simulink library "halout"  (R2021b)
settings: Solver=VariableStepAuto  StartTime=0.0  StopTime=10.0  RelTol=1e-3
undefined symbols (not defined in the file): C_TASK_5MS_S, FALSE, KHAL_CAN1FD1APS3E2E_flg, KHAL_CAN1FD1APS3TxReq_flg, KHAL_CAN1FD1VCU2E2E_flg, KHAL_CAN1FD1VCU2TxReq_flg, KHAL_CAN1FD1VCU3E2E_flg, KHAL_CAN1FD1VCU3TxReq_flg, KHAL_CAN1TxReq_flg, KHAL_CAN1VMCFCM1E2E_flg, KHAL_CAN1VMCFCM1TxReq_flg, KHAL_CAN2TxReq_flg, KHAL_CAN3FD3VCU1toNIDECTxReq_flg, KHAL_CAN3FD3VCU1TxReq_flg, KHAL_CAN3FD3VCU2E2E_flg, KHAL_CAN3FD3VCU2toNIDECE2E_flg, KHAL_CAN3FD3VCU2toNIDECTxReq_flg, KHAL_CAN3FD3VCU2TxReq_flg, KHAL_CAN3TxReq_flg, KHAL_CAN4FD4CE1000E2E_flg, KHAL_CAN4FD4CE1000TxReq_flg, KHAL_CAN4TxReq_flg, KHAL_CAN5TxReq_flg, KHAL_CAN6FD6APS3E2E_flg, KHAL_CAN6FD6APS3TxReq_flg, KHAL_CAN6FD6VCU2E2E_flg, KHAL_CAN6FD6VCU2TxReq_flg, KHAL_CAN6TxReq_flg, ONE_INT, TRUE, ZERO_INT
libraries: FVT_lib x551, simulink x244
(part 9 of 26)

== system halout/HAL_OUT/CAN3/FD3_VCU5_0x155 ==
  BSCP_outputs : Inport  OutDataTypeStr=Bus: BSCP_outputs
  BOUTP_outputs : Inport  Port=2  OutDataTypeStr=Bus: BOUTP_outputs
  ActAPSPosn : Subsystem
  FDCVCUFrSpdMaxReq : Subsystem
  FDCVCUFrSpdMinReq : Subsystem
  FDCVCUFrTMCtrlModeReq : Subsystem
  FDCVCUFrTMSpdReq : Subsystem
  FDCVCUFrTMTqReq : Subsystem
  FDCVCUFrTqMaxReq : Subsystem
  FDCVCUFrTqMinReq : Subsystem
  FDCVCURrSpdMaxReq : Subsystem
  FDCVCURrSpdMinReq : Subsystem
  FDCVCURrTMCtrlModeReq : Subsystem
  FDCVCURrTMSpdReq : Subsystem
  FDCVCURrTMTqReq : Subsystem
  FDCVCURrTqMaxReq : Subsystem
  FDCVCURrTqMinReq : Subsystem
  FrEDUSpd : Subsystem
  FrEDUSpdValid : Subsystem
  Ground{,1..13} (14 alike) : Ground
  RrEDUSpd : Subsystem
  RrEDUSpdValid : Subsystem
  bus_creator : BusCreator  Inputs=19  OutDataTypeStr=Bus: DT_CAN3_SG_FD3_VCU5  NonVirtualBus=on
  bus_selector : BusSelector  OutputSignals=VOUTP_ActAPSPosn_pct
  bus_selector1 : BusSelector  OutputSignals=VOUTP_FrEDUSpd_rpm
  bus_selector2 : BusSelector  OutputSignals=VOUTP_FrEDUSpdValid_flg
  bus_selector3 : BusSelector  OutputSignals=VOUTP_RrEDUSpd_rpm
  bus_selector4 : BusSelector  OutputSignals=VOUTP_RrEDUSpdValid_flg
  FD3_VCU5 : Outport
  wires:
  BSCP_outputs/1 -> [BSCP_outputs]
  BOUTP_outputs/1 -> [BOUTP_outputs]
  [CAN3_ActAPSPosn] -> bus_creator/1  "CAN3_ActAPSPosn"
  [CAN3_FDC_VCU_FrSpdMax_Req] -> bus_creator/2  "CAN3_FDC_VCU_FrSpdMax_Req"
  [CAN3_FDC_VCU_FrSpdMin_Req] -> bus_creator/3  "CAN3_FDC_VCU_FrSpdMin_Req"
  [CAN3_FDC_VCU_FrTMCtrlMode_Req] -> bus_creator/4  "CAN3_FDC_VCU_FrTMCtrlMode_Req"
  [CAN3_FDC_VCU_FrTMSpd_Req] -> bus_creator/5  "CAN3_FDC_VCU_FrTMSpd_Req"
  [CAN3_FDC_VCU_FrTMTq_Req] -> bus_creator/6  "CAN3_FDC_VCU_FrTMTq_Req"
  [CAN3_FDC_VCU_FrTqMax_Req] -> bus_creator/7  "CAN3_FDC_VCU_FrTqMax_Req"
  [CAN3_FDC_VCU_FrTqMin_Req] -> bus_creator/8  "CAN3_FDC_VCU_FrTqMin_Req"
  [CAN3_FDC_VCU_RrSpdMax_Req] -> bus_creator/9  "CAN3_FDC_VCU_RrSpdMax_Req"
  [CAN3_FDC_VCU_RrSpdMin_Req] -> bus_creator/10  "CAN3_FDC_VCU_RrSpdMin_Req"
  [CAN3_FDC_VCU_RrTMCtrlMode_Req] -> bus_creator/11  "CAN3_FDC_VCU_RrTMCtrlMode_Req"
  [CAN3_FDC_VCU_RrTMSpd_Req] -> bus_creator/12  "CAN3_FDC_VCU_RrTMSpd_Req"
  [CAN3_FDC_VCU_RrTMTq_Req] -> bus_creator/13  "CAN3_FDC_VCU_RrTMTq_Req"
  [CAN3_FDC_VCU_RrTqMax_Req] -> bus_creator/14  "CAN3_FDC_VCU_RrTqMax_Req"
  [CAN3_FDC_VCU_RrTqMin_Req] -> bus_creator/15  "CAN3_FDC_VCU_RrTqMin_Req"
  [CAN3_Fr_EDUSpd] -> bus_creator/16  "CAN3_Fr_EDUSpd"
  [CAN3_Fr_EDUSpdValid] -> bus_creator/17  "CAN3_Fr_EDUSpdValid"
  [CAN3_Rr_EDUSpd] -> bus_creator/18  "CAN3_Rr_EDUSpd"
  [CAN3_Rr_EDUSpdValid] -> bus_creator/19  "CAN3_Rr_EDUSpdValid"
  bus_creator/1 -> FD3_VCU5/1
  ActAPSPosn/1(CAN3_ActAPSPosn) -> [CAN3_ActAPSPosn]
  FDCVCUFrSpdMaxReq/1(CAN3_FDC_VCU_FrSpdMax_Req) -> [CAN3_FDC_VCU_FrSpdMax_Req]
  FDCVCUFrSpdMinReq/1(CAN3_FDC_VCU_FrSpdMin_Req) -> [CAN3_FDC_VCU_FrSpdMin_Req]
  FDCVCUFrTMCtrlModeReq/1(CAN3_FDC_VCU_FrTMCtrlMode_Req) -> [CAN3_FDC_VCU_FrTMCtrlMode_Req]
  FDCVCUFrTMSpdReq/1(CAN3_FDC_VCU_FrTMSpd_Req) -> [CAN3_FDC_VCU_FrTMSpd_Req]
  FDCVCUFrTMTqReq/1(CAN3_FDC_VCU_FrTMTq_Req) -> [CAN3_FDC_VCU_FrTMTq_Req]
  FDCVCUFrTqMaxReq/1(CAN3_FDC_VCU_FrTqMax_Req) -> [CAN3_FDC_VCU_FrTqMax_Req]
  FDCVCUFrTqMinReq/1(CAN3_FDC_VCU_FrTqMin_Req) -> [CAN3_FDC_VCU_FrTqMin_Req]
  FDCVCURrSpdMaxReq/1(CAN3_FDC_VCU_RrSpdMax_Req) -> [CAN3_FDC_VCU_RrSpdMax_Req]
  FDCVCURrSpdMinReq/1(CAN3_FDC_VCU_RrSpdMin_Req) -> [CAN3_FDC_VCU_RrSpdMin_Req]
  FDCVCURrTMCtrlModeReq/1(CAN3_FDC_VCU_RrTMCtrlMode_Req) -> [CAN3_FDC_VCU_RrTMCtrlMode_Req]
  FDCVCURrTMSpdReq/1(CAN3_FDC_VCU_RrTMSpd_Req) -> [CAN3_FDC_VCU_RrTMSpd_Req]
  FDCVCURrTMTqReq/1(CAN3_FDC_VCU_RrTMTq_Req) -> [CAN3_FDC_VCU_RrTMTq_Req]
  FDCVCURrTqMaxReq/1(CAN3_FDC_VCU_RrTqMax_Req) -> [CAN3_FDC_VCU_RrTqMax_Req]
  FDCVCURrTqMinReq/1(CAN3_FDC_VCU_RrTqMin_Req) -> [CAN3_FDC_VCU_RrTqMin_Req]
  FrEDUSpd/1(CAN3_Fr_EDUSpd) -> [CAN3_Fr_EDUSpd]
  FrEDUSpdValid/1(CAN3_Fr_EDUSpdValid) -> [CAN3_Fr_EDUSpdValid]
  RrEDUSpd/1(CAN3_Rr_EDUSpd) -> [CAN3_Rr_EDUSpd]
  RrEDUSpdValid/1(CAN3_Rr_EDUSpdValid) -> [CAN3_Rr_EDUSpdValid]
  bus_selector/1 -> ActAPSPosn/1(ActAPSPosn)  "<VOUTP_ActAPSPosn_pct>"
  [BOUTP_outputs] -> bus_selector/1
  Ground/1 -> FDCVCUFrSpdMaxReq/1(FDCVCUFrSpdMaxReq)
  Ground1/1 -> FDCVCUFrSpdMinReq/1(FDCVCUFrSpdMinReq)
  Ground2/1 -> FDCVCUFrTMCtrlModeReq/1(FDCVCUFrTMCtrlModeReq)
  Ground3/1 -> FDCVCUFrTMSpdReq/1(FDCVCUFrTMSpdReq)
  Ground4/1 -> FDCVCUFrTMTqReq/1(FDCVCUFrTMTqReq)
  Ground5/1 -> FDCVCUFrTqMaxReq/1(FDCVCUFrTqMaxReq)
  Ground6/1 -> FDCVCUFrTqMinReq/1(FDCVCUFrTqMinReq)
  Ground7/1 -> FDCVCURrSpdMaxReq/1(FDCVCURrSpdMaxReq)
  Ground8/1 -> FDCVCURrSpdMinReq/1(FDCVCURrSpdMinReq)
  Ground9/1 -> FDCVCURrTMCtrlModeReq/1(FDCVCURrTMCtrlModeReq)
  Ground10/1 -> FDCVCURrTMSpdReq/1(FDCVCURrTMSpdReq)
  Ground11/1 -> FDCVCURrTMTqReq/1(FDCVCURrTMTqReq)
  Ground12/1 -> FDCVCURrTqMaxReq/1(FDCVCURrTqMaxReq)
  Ground13/1 -> FDCVCURrTqMinReq/1(FDCVCURrTqMinReq)
  bus_selector1/1 -> FrEDUSpd/1(FrEDUSpd)  "<VOUTP_FrEDUSpd_rpm>"
  [BOUTP_outputs] -> bus_selector1/1
  bus_selector2/1 -> FrEDUSpdValid/1(FrEDUSpdValid)  "<VOUTP_FrEDUSpdValid_flg>"
  [BOUTP_outputs] -> bus_selector2/1
  bus_selector3/1 -> RrEDUSpd/1(RrEDUSpd)  "<VOUTP_RrEDUSpd_rpm>"
  [BOUTP_outputs] -> bus_selector3/1
  bus_selector4/1 -> RrEDUSpdValid/1(RrEDUSpdValid)  "<VOUTP_RrEDUSpdValid_flg>"
  [BOUTP_outputs] -> bus_selector4/1

== system halout/HAL_OUT/CAN3/GW_ESC1_toNIDEC_0x152 ==
  BSCP_outputs : Inport  OutDataTypeStr=Bus: BSCP_outputs
  BOUTP_outputs : Inport  Port=2  OutDataTypeStr=Bus: BOUTP_outputs
  VehSpeedtoNidec : Subsystem
  bus_creator : BusCreator  Inputs=1  OutDataTypeStr=Bus: DT_CAN3_SG_GW_ESC1_toNIDEC  NonVirtualBus=on
  bus_selector : BusSelector  OutputSignals=VSCP_CAN3GWESC1toNIDECVehSpeedtoNidec_kph
  GW_ESC1_toNIDEC : Outport
  wires:
  BSCP_outputs/1 -> [BSCP_outputs]
  BOUTP_outputs/1 -> [BOUTP_outputs]
  [CAN3_VehSpeed_toNidec] -> bus_creator/1  "CAN3_VehSpeed_toNidec"
  bus_creator/1 -> GW_ESC1_toNIDEC/1
  VehSpeedtoNidec/1(CAN3_VehSpeed_toNidec) -> [CAN3_VehSpeed_toNidec]
  bus_selector/1 -> VehSpeedtoNidec/1(VehSpeedtoNidec)  "<VSCP_CAN3GWESC1toNIDECVehSpeedtoNidec_kph>"
  [BSCP_outputs] -> bus_selector/1

== system halout/HAL_OUT/CAN3/GW_IVI6_toNIDEC_0x49F ==
  BSCP_outputs : Inport  OutDataTypeStr=Bus: BSCP_outputs
  BOUTP_outputs : Inport  Port=2  OutDataTypeStr=Bus: BOUTP_outputs
  IVITimeDaytoNidec : Subsystem
  IVITimeHourtoNidec : Subsystem
  IVITimeMinutetoNidec : Subsystem
  IVITimeMonthtoNidec : Subsystem
  IVITimeSecondtoNidec : Subsystem
  bus_creator : BusCreator  Inputs=5  OutDataTypeStr=Bus: DT_CAN3_SG_GW_IVI6_toNIDEC  NonVirtualBus=on
  bus_selector : BusSelector  OutputSignals=VSCP_CAN3GWIVI6toNIDECIVITimeDaytoNidec_DAY
  bus_selector1 : BusSelector  OutputSignals=VSCP_CAN3GWIVI6toNIDECIVITimeHourtoNidec_hr
  bus_selector2 : BusSelector  OutputSignals=VSCP_CAN3GWIVI6toNIDECIVITimeMinutetoNidec_min
  bus_selector3 : BusSelector  OutputSignals=VSCP_CAN3GWIVI6toNIDECIVITimeMonthtoNidec_MONTH
  bus_selector4 : BusSelector  OutputSignals=VSCP_CAN3GWIVI6toNIDECIVITimeSecondtoNidec_s
  GW_IVI6_toNIDEC : Outport
  wires:
  BSCP_outputs/1 -> [BSCP_outputs]
  BOUTP_outputs/1 -> [BOUTP_outputs]
  [CAN3_IVI_Time_Day_toNidec] -> bus_creator/1  "CAN3_IVI_Time_Day_toNidec"
  [CAN3_IVI_Time_Hour_toNidec] -> bus_creator/2  "CAN3_IVI_Time_Hour_toNidec"
  [CAN3_IVI_Time_Minute_toNidec] -> bus_creator/3  "CAN3_IVI_Time_Minute_toNidec"
  [CAN3_IVI_Time_Month_toNidec] -> bus_creator/4  "CAN3_IVI_Time_Month_toNidec"
  [CAN3_IVI_Time_Second_toNidec] -> bus_creator/5  "CAN3_IVI_Time_Second_toNidec"
  bus_creator/1 -> GW_IVI6_toNIDEC/1
  IVITimeDaytoNidec/1(CAN3_IVI_Time_Day_toNidec) -> [CAN3_IVI_Time_Day_toNidec]
  IVITimeHourtoNidec/1(CAN3_IVI_Time_Hour_toNidec) -> [CAN3_IVI_Time_Hour_toNidec]
  IVITimeMinutetoNidec/1(CAN3_IVI_Time_Minute_toNidec) -> [CAN3_IVI_Time_Minute_toNidec]
  IVITimeMonthtoNidec/1(CAN3_IVI_Time_Month_toNidec) -> [CAN3_IVI_Time_Month_toNidec]
  IVITimeSecondtoNidec/1(CAN3_IVI_Time_Second_toNidec) -> [CAN3_IVI_Time_Second_toNidec]
  bus_selector/1 -> IVITimeDaytoNidec/1(IVITimeDaytoNidec)  "<VSCP_CAN3GWIVI6toNIDECIVITimeDaytoNidec_DAY>"
  [BSCP_outputs] -> bus_selector/1
  bus_selector1/1 -> IVITimeHourtoNidec/1(IVITimeHourtoNidec)  "<VSCP_CAN3GWIVI6toNIDECIVITimeHourtoNidec_hr>"
  [BSCP_outputs] -> bus_selector1/1
  bus_selector2/1 -> IVITimeMinutetoNidec/1(IVITimeMinutetoNidec)  "<VSCP_CAN3GWIVI6toNIDECIVITimeMinutetoNidec_min>"
  [BSCP_outputs] -> bus_selector2/1
  bus_selector3/1 -> IVITimeMonthtoNidec/1(IVITimeMonthtoNidec)  "<VSCP_CAN3GWIVI6toNIDECIVITimeMonthtoNidec_MONTH>"
  [BSCP_outputs] -> bus_selector3/1
  bus_selector4/1 -> IVITimeSecondtoNidec/1(IVITimeSecondtoNidec)  "<VSCP_CAN3GWIVI6toNIDECIVITimeSecondtoNidec_s>"
  [BSCP_outputs] -> bus_selector4/1

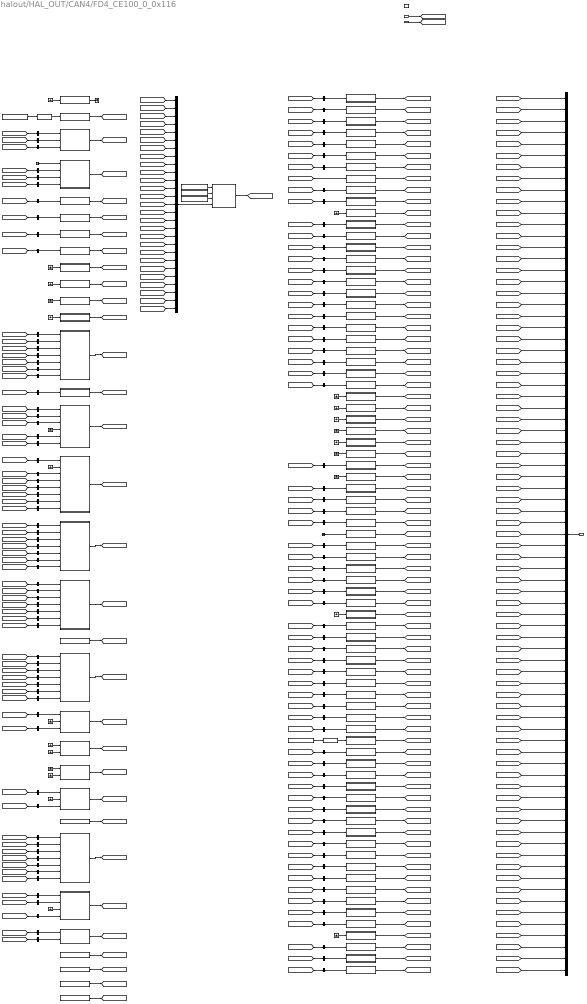
== system halout/HAL_OUT/CAN4/FD4_CE100_0_0x116 ==
  BSCP_outputs : Inport  OutDataTypeStr=Bus: BSCP_outputs
  BOUTP_outputs : Inport  Port=2  OutDataTypeStr=Bus: BOUTP_outputs
  Trigger : TriggerPort  TriggerType=function-call  VariantControl=(inherit)
  APSStaSystem : Subsystem
  AllDoorSW : Subsystem
  AntiTheftSeatFold : Subsystem
  AntitheftSta : Subsystem
  BCMDoorLockSta : Subsystem
  BrakeLamp : Subsystem
  Byte_0 : Subsystem
  Byte_1 : Subsystem
  Byte_10 : Subsystem
  Byte_11 : Subsystem
  Byte_12 : Subsystem
  Byte_13 : Subsystem
  Byte_14 : Subsystem
  Byte_15 : Subsystem
  Byte_16 : Subsystem
  Byte_17 : Subsystem
  Byte_{18,24,28..31} (6 alike) : Constant  Value=ZERO_INT
  Byte_19 : Subsystem
  Byte_2 : Subsystem
  Byte_20 : Subsystem
  Byte_21 : Subsystem
  Byte_22 : Subsystem
  Byte_23 : Subsystem
  Byte_25 : Subsystem
  Byte_26 : Subsystem
  Byte_27 : Subsystem
  Byte_3 : Subsystem
  Byte_4 : Subsystem
  Byte_5 : Subsystem
  Byte_6 : Subsystem
  Byte_7 : Subsystem
  Byte_8 : Subsystem
  Byte_9 : Subsystem
  CCCrlSta : Subsystem
  CRC8_IfAction_Tx : Subsystem  AncestorBlock=FVT_lib/hal/CRC8_IfAction_Tx
      mask help: MeasumentTrigerEvent
      mask Display: fprintf('CRC8_IfAction');
  CSVCU1CAN4 : Subsystem
  CTDCtrl : Subsystem
  CTDLockSW : Subsystem
  CTDUnlockSW : Subsystem
  Constant : Constant  Value=KHAL_CAN4FD4CE1000E2E_flg
  Constant1 : Constant  Value=0x08
  Constant2 : Constant  Value=0x4D
  Constant3 : Constant  Value=KHAL_CAN4FD4CE1000E2E_flg
  Constant4 : Constant  Value=KHAL_CAN4FD4CE1000E2E_flg
  CrashDetd : Subsystem
  CtrlDrPwrStbA2 : Subsystem
  CtrlFrBMSCCUCIR : Subsystem
  CtrlFrEDUINVERTER : Subsystem
  CtrlFrIRC1 : Subsystem
  CtrlFrPwrStbA1P : Subsystem
  DKCAuthSta : Subsystem
  DKCTimeSN : Subsystem
  Dimmer : Subsystem
  DimmerEN : Subsystem
  DoorLockIND : Subsystem
  DrDoorSW : Subsystem
  DrSeatSta : Subsystem
  EquivAccPedalSWSta : Subsystem
  FDCVMCVehPitchAngleSta : Subsystem
  FDDKCVehDataErr : Subsystem
  FDDKCVehDataSta : Subsystem
  FDTBOXDTCDataErr : Subsystem
  FDTBOXDTCDataSta : Subsystem
  FDTBOXVehDataErr : Subsystem
  FDTBOXVehDataSta : Subsystem
  FrChargingDoorCtrl : Subsystem
  FrFogLamp : Subsystem
  FrWiperH : Subsystem
  FrWiperL : Subsystem
  Ground{,1..25} (26 alike) : Ground
  HBeam : Subsystem
  HBeamADB : Subsystem
  HWResetSta : Subsystem
  HazardSW : Subsystem
  HoodSW : Subsystem
  HornCtrl : Subsystem
  LAPMWdwEnable : Subsystem
  LBSD : Subsystem
  LBeam : Subsystem
  LDRL : Subsystem
  LTurnLP : Subsystem
  LampPwr : Subsystem
  LockSetting : Subsystem
  MSACrlSta : Subsystem
  MirrorCtrl : Subsystem
  MirrorDefog : Subsystem
  Mux2 : Mux  Inputs=27
  PosLamp : Subsystem
  PsDoorSW : Subsystem
  PwrSta : Subsystem
  RBSD : Subsystem
  RCVCU1CAN4 : Subsystem
  RDRL : Subsystem
  RLDoorSW : Subsystem
  RRDoorSW : Subsystem
  RTurnLP : Subsystem
  ReBrakeLPReq : Subsystem
  ReverseLamp : Subsystem
  RollingCounter_IfAction : FVT_lib/hal/RollingCounter_IfAction
  RollingCounter_IfAction1 : FVT_lib/hal/RollingCounter_IfAction
  RoomLampH : Subsystem
  RoomLampL : Subsystem
  RrChargingDoorCtrl : Subsystem
  RrDefog : Subsystem
  RrFogLamp : Subsystem
  RrWiper : Subsystem
  ShiftGearPosn : Subsystem
  TailgateHDSW : Subsystem
  TailgateRemote : Subsystem
  TailgateSW : Subsystem
  Terminator : Terminator
  TimeSNDKCFbk : Subsystem
  TrunkRel : Subsystem
  WasherCtrl : Subsystem
  WiperFixMode : Subsystem
  bus_creator : BusCreator  Inputs=77  OutDataTypeStr=Bus: DT_CAN4_SG_FD4_CE100_0  NonVirtualBus=on
  bus_selector : BusSelector  OutputSignals=VOUTP_CCCtrlSta_enum
  bus_selector1 : BusSelector  OutputSignals=VOUTP_DrSeatSta_enum
  bus_selector{7..10,84} (5 alike) : BusSelector  OutputSignals=VOUTP_DKCTimeSN_cnt
  bus_selector100 : BusSelector  OutputSignals=VOUTP_HornCtrl_flg
  bus_selector101 : BusSelector  OutputSignals=VOUTP_LBSD_flg
  bus_selector102 : BusSelector  OutputSignals=VOUTP_LDRL_flg
  bus_selector103 : BusSelector  OutputSignals=VOUTP_LTurnLP_flg
  bus_selector104 : BusSelector  OutputSignals=VOUTP_LBeam_flg
  bus_selector105 : BusSelector  OutputSignals=VOUTP_LampPwr_flg
  bus_selector106 : BusSelector  OutputSignals=VOUTP_LockSetting_flg
  bus_selector107 : BusSelector  OutputSignals=VOUTP_MSACtrlSta_enum
  bus_selector108 : BusSelector  OutputSignals=VOUTP_MirrorCtrl_enum
  bus_selector109 : BusSelector  OutputSignals=VOUTP_MirrorDefog_flg
  bus_selector11 : BusSelector  OutputSignals=VOUTP_BCMDoorLockSta_flg
  bus_selector110 : BusSelector  OutputSignals=VOUTP_PosLamp_flg
  bus_selector111 : BusSelector  OutputSignals=VOUTP_PsDoorSW_flg
  bus_selector112 : BusSelector  OutputSignals=VOUTP_PowerSta_enum
  bus_selector113 : BusSelector  OutputSignals=VOUTP_RBSD_flg
  bus_selector114 : BusSelector  OutputSignals=VOUTP_RDRL_flg
  bus_selector115 : BusSelector  OutputSignals=VOUTP_RLDoorSW_flg
  bus_selector116 : BusSelector  OutputSignals=VOUTP_RRDoorSW_flg
  bus_selector117 : BusSelector  OutputSignals=VOUTP_RTurnLP_flg
  bus_selector118 : BusSelector  OutputSignals=VOUTP_ReBrakeLPReq_flg
  bus_selector119 : BusSelector  OutputSignals=VOUTP_ReverseLamp_flg
  bus_selector12 : BusSelector  OutputSignals=VOUTP_DimmerEN_flg
  bus_selector120 : BusSelector  OutputSignals=VOUTP_RoomLampH_flg
  bus_selector121 : BusSelector  OutputSignals=VOUTP_RoomLampL_flg
  bus_selector122 : BusSelector  OutputSignals=VOUTP_RrChargingDoorCtrl_enum
  bus_selector123 : BusSelector  OutputSignals=VOUTP_RrDefog_flg
  bus_selector124 : BusSelector  OutputSignals=VOUTP_RrFogLamp_flg
  bus_selector125 : BusSelector  OutputSignals=VOUTP_RrWiper_flg
  bus_selector126 : BusSelector  OutputSignals=VOUTP_ShiftGearPosn_enum
  bus_selector127 : BusSelector  OutputSignals=VOUTP_TailgateHDSW_flg
  bus_selector128 : BusSelector  OutputSignals=VOUTP_TailgateRemote_enum
  bus_selector129 : BusSelector  OutputSignals=VOUTP_TailgateSW_flg
  bus_selector13 : BusSelector  OutputSignals=VOUTP_EquivAccPedalSWSta_flg
  bus_selector130 : BusSelector  OutputSignals=VOUTP_TrunkRel_flg
  bus_selector131 : BusSelector  OutputSignals=VOUTP_WasherCtrl_enum
  bus_selector132 : BusSelector  OutputSignals=VOUTP_WiperFixMode_flg
  bus_selector14 : BusSelector  OutputSignals=VOUTP_HornCtrl_flg
  bus_selector15 : BusSelector  OutputSignals=VOUTP_RoomLampH_flg
  bus_selector16 : BusSelector  OutputSignals=VOUTP_RoomLampL_flg
  bus_selector17 : BusSelector  OutputSignals=VOUTP_TailgateRemote_enum
  bus_selector18 : BusSelector  OutputSignals=VOUTP_Dimmer_pct
  bus_selector19 : BusSelector  OutputSignals=VOUTP_AntitheftSeatFlod_flg
  bus_selector2 : BusSelector  OutputSignals=VOUTP_MSACtrlSta_enum
  bus_selector20 : BusSelector  OutputSignals=VOUTP_AntitheftSta_enum
  bus_selector21 : BusSelector  OutputSignals=VOUTP_CrashDetd_flg
  bus_selector22 : BusSelector  OutputSignals=VOUTP_LockSetting_flg
  bus_selector23 : BusSelector  OutputSignals=VOUTP_RTurnLP_flg
  bus_selector24 : BusSelector  OutputSignals=VOUTP_BrakeLamp_flg
  bus_selector25 : BusSelector  OutputSignals=VOUTP_HazardSW_flg
  bus_selector26 : BusSelector  OutputSignals=VOUTP_LBSD_flg
  bus_selector27 : BusSelector  OutputSignals=VOUTP_LTurnLP_flg
  bus_selector28 : BusSelector  OutputSignals=VOUTP_RBSD_flg
  bus_selector29 : BusSelector  OutputSignals=VOUTP_ReverseLamp_flg
  bus_selector30 : BusSelector  OutputSignals=VOUTP_RrFogLamp_flg
  bus_selector31 : BusSelector  OutputSignals=VOUTP_HBeam_flg
  bus_selector32 : BusSelector  OutputSignals=VOUTP_LDRL_flg
  bus_selector33 : BusSelector  OutputSignals=VOUTP_LBeam_flg
  bus_selector34 : BusSelector  OutputSignals=VOUTP_PosLamp_flg
  bus_selector35 : BusSelector  OutputSignals=VOUTP_RDRL_flg
  bus_selector36 : BusSelector  OutputSignals=VOUTP_WasherCtrl_enum
  bus_selector37 : BusSelector  OutputSignals=VOUTP_WiperFixMode_flg
  bus_selector38 : BusSelector  OutputSignals=VOUTP_FrWiperH_flg
  bus_selector39 : BusSelector  OutputSignals=VOUTP_FrWiperL_flg
  bus_selector4 : BusSelector  OutputSignals=VOUTP_PowerSta_enum
  bus_selector40 : BusSelector  OutputSignals=VOUTP_MirrorCtrl_enum
  bus_selector41 : BusSelector  OutputSignals=VOUTP_RrDefog_flg
  bus_selector42 : BusSelector  OutputSignals=VOUTP_RrWiper_flg
  bus_selector43 : BusSelector  OutputSignals=VOUTP_TailgateHDSW_flg
  bus_selector44 : BusSelector  OutputSignals=VOUTP_TrunkRel_flg
  bus_selector45 : BusSelector  OutputSignals=VOUTP_AllDoorSW_flg
  bus_selector46 : BusSelector  OutputSignals=VOUTP_DoorLockIND_flg
  bus_selector47 : BusSelector  OutputSignals=VOUTP_FrChargingDoorCtrl_enum
  bus_selector48 : BusSelector  OutputSignals=VOUTP_HoodSW_flg
  bus_selector49 : BusSelector  OutputSignals=VOUTP_PsDoorSW_flg
  bus_selector5 : BusSelector  OutputSignals=VOUTP_ReBrakeLPReq_flg
  bus_selector50 : BusSelector  OutputSignals=VOUTP_RLDoorSW_flg
  bus_selector51 : BusSelector  OutputSignals=VOUTP_RRDoorSW_flg
  bus_selector52 : BusSelector  OutputSignals=VOUTP_CTDCtrl_enum
  bus_selector53 : BusSelector  OutputSignals=VOUTP_RrChargingDoorCtrl_enum
  bus_selector54 : BusSelector  OutputSignals=VOUTP_DKCAuthSta_enum
  bus_selector55 : BusSelector  OutputSignals=VOUTP_LampPwr_flg
  bus_selector56 : BusSelector  OutputSignals=VOUTP_CtrlFrBMSCCUCIR_flg
  bus_selector57 : BusSelector  OutputSignals=VOUTP_CtrlFrEDUINVERTER_flg
  bus_selector58 : BusSelector  OutputSignals=VOUTP_CtrlFrRC1_flg
  bus_selector59 : BusSelector  OutputSignals=VOUTP_CtrlFrPwrStbA1P_flg
  bus_selector6 : BusSelector  OutputSignals=VOUTP_ShiftGearPosn_enum
  bus_selector60 : BusSelector  OutputSignals=VOUTP_DrDoorSW_flg
  bus_selector61 : BusSelector  OutputSignals=VOUTP_HWResetSta_enum
  bus_selector62 : BusSelector  OutputSignals=VOUTP_MirrorDefog_flg
  bus_selector63 : BusSelector  OutputSignals=VOUTP_APSStaSys_enum
  bus_selector64 : BusSelector  OutputSignals=VOUTP_CTDLockSW_flg
  bus_selector65 : BusSelector  OutputSignals=VOUTP_VehPitchAngleSta_enum
  bus_selector66 : BusSelector  OutputSignals=VOUTP_CtrlDrPwrStbA2_flg
  bus_selector67 : BusSelector  OutputSignals=VOUTP_TailgateSW_flg
  bus_selector68 : BusSelector  OutputSignals=VOUTP_APSStaSys_enum
  bus_selector69 : BusSelector  OutputSignals=VOUTP_AllDoorSW_flg
  bus_selector70 : BusSelector  OutputSignals=VOUTP_AntitheftSeatFlod_flg
  bus_selector71 : BusSelector  OutputSignals=VOUTP_AntitheftSta_enum
  bus_selector72 : BusSelector  OutputSignals=VOUTP_BCMDoorLockSta_flg
  bus_selector73 : BusSelector  OutputSignals=VOUTP_BrakeLamp_flg
  bus_selector74 : BusSelector  OutputSignals=VOUTP_CCCtrlSta_enum
  bus_selector75 : BusSelector  OutputSignals=VOUTP_CTDCtrl_enum
  bus_selector76 : BusSelector  OutputSignals=VOUTP_CTDLockSW_flg
  bus_selector77 : BusSelector  OutputSignals=VOUTP_CrashDetd_flg
  bus_selector78 : BusSelector  OutputSignals=VOUTP_CtrlDrPwrStbA2_flg
  bus_selector79 : BusSelector  OutputSignals=VOUTP_CtrlFrBMSCCUCIR_flg
  bus_selector80 : BusSelector  OutputSignals=VOUTP_CtrlFrEDUINVERTER_flg
  bus_selector81 : BusSelector  OutputSignals=VOUTP_CtrlFrRC1_flg
  bus_selector82 : BusSelector  OutputSignals=VOUTP_CtrlFrPwrStbA1P_flg
  bus_selector83 : BusSelector  OutputSignals=VOUTP_DKCAuthSta_enum
  bus_selector85 : BusSelector  OutputSignals=VOUTP_Dimmer_pct
  bus_selector86 : BusSelector  OutputSignals=VOUTP_DimmerEN_flg
  bus_selector87 : BusSelector  OutputSignals=VOUTP_DoorLockIND_flg
  bus_selector88 : BusSelector  OutputSignals=VOUTP_DrDoorSW_flg
  bus_selector89 : BusSelector  OutputSignals=VOUTP_DrSeatSta_enum
  bus_selector90 : BusSelector  OutputSignals=VOUTP_EquivAccPedalSWSta_flg
  bus_selector91 : BusSelector  OutputSignals=VOUTP_VehPitchAngleSta_enum
  bus_selector92 : BusSelector  OutputSignals=VOUTP_FrChargingDoorCtrl_enum
  bus_selector93 : BusSelector  OutputSignals=VOUTP_FrWiperH_flg
  bus_selector94 : BusSelector  OutputSignals=VOUTP_FrWiperL_flg
  bus_selector95 : BusSelector  OutputSignals=VOUTP_HWResetSta_enum
  bus_selector96 : BusSelector  OutputSignals=VOUTP_HBeam_flg
  bus_selector98 : BusSelector  OutputSignals=VOUTP_HazardSW_flg
  bus_selector99 : BusSelector  OutputSignals=VOUTP_HoodSW_flg
  FD4_CE100_0 : Outport
  wires:
  BSCP_outputs/1 -> [BSCP_outputs]
  BOUTP_outputs/1 -> [BOUTP_outputs]
  [CAN4_APS_Sta_System] -> bus_creator/1  "CAN4_APS_Sta_System"
  [CAN4_AllDoorSW] -> bus_creator/2  "CAN4_AllDoorSW"
  [CAN4_AntiTheftSeatFold] -> bus_creator/3  "CAN4_AntiTheftSeatFold"
  [CAN4_AntitheftSta] -> bus_creator/4  "CAN4_AntitheftSta"
  [CAN4_BCM_DoorLock_Sta] -> bus_creator/5  "CAN4_BCM_DoorLock_Sta"
  [CAN4_BrakeLamp] -> bus_creator/6  "CAN4_BrakeLamp"
  [CAN4_CC_Crl_Sta] -> bus_creator/7  "CAN4_CC_Crl_Sta"
  [CAN4_CS_VCU1_CAN4] -> bus_creator/8  "CAN4_CS_VCU1_CAN4"
  [CAN4_CTDCtrl] -> bus_creator/9  "CAN4_CTDCtrl"
  [CAN4_CTDLockSW] -> bus_creator/10  "CAN4_CTDLockSW"
  [CAN4_CTDUnlockSW] -> bus_creator/11  "CAN4_CTDUnlockSW"
  [CAN4_CrashDetd] -> bus_creator/12  "CAN4_CrashDetd"
  [CAN4_CtrlDrPwrStbA2] -> bus_creator/13  "CAN4_CtrlDrPwrStbA2"
  [CAN4_CtrlFrBMSCCUCIR] -> bus_creator/14  "CAN4_CtrlFrBMSCCUCIR"
  [CAN4_CtrlFrEDUINVERTER] -> bus_creator/15  "CAN4_CtrlFrEDUINVERTER"
  [CAN4_CtrlFrIRC1] -> bus_creator/16  "CAN4_CtrlFrIRC1"
  [CAN4_CtrlFrPwrStbA1P] -> bus_creator/17  "CAN4_CtrlFrPwrStbA1P"
  [CAN4_DKCAuthSta] -> bus_creator/18  "CAN4_DKCAuthSta"
  [CAN4_DKCTimeSN] -> bus_creator/19  "CAN4_DKCTimeSN"
  [CAN4_Dimmer] -> bus_creator/20  "CAN4_Dimmer"
  [CAN4_DimmerEN] -> bus_creator/21  "CAN4_DimmerEN"
  [CAN4_DoorLockIND] -> bus_creator/22  "CAN4_DoorLockIND"
  [CAN4_DrDoorSW] -> bus_creator/23  "CAN4_DrDoorSW"
  [CAN4_Dr_SeatSta] -> bus_creator/24  "CAN4_Dr_SeatSta"
  [CAN4_EquivAccPedalSWSta] -> bus_creator/25  "CAN4_EquivAccPedalSWSta"
  [CAN4_FDC_VMC_VehPitchAngle_Sta] -> bus_creator/26  "CAN4_FDC_VMC_VehPitchAngle_Sta"
  [CAN4_FD_DKC_VehData_Err] -> bus_creator/27  "CAN4_FD_DKC_VehData_Err"
  [CAN4_FD_DKC_VehData_Sta] -> bus_creator/28  "CAN4_FD_DKC_VehData_Sta"
  [CAN4_FD_TBOX_DTCData_Err] -> bus_creator/29  "CAN4_FD_TBOX_DTCData_Err"
  [CAN4_FD_TBOX_DTCData_Sta] -> bus_creator/30  "CAN4_FD_TBOX_DTCData_Sta"
  [CAN4_FD_TBOX_VehData_Err] -> bus_creator/31  "CAN4_FD_TBOX_VehData_Err"
  [CAN4_FD_TBOX_VehData_Sta] -> bus_creator/32  "CAN4_FD_TBOX_VehData_Sta"
  [CAN4_Fr_ChargingDoorCtrl] -> bus_creator/33  "CAN4_Fr_ChargingDoorCtrl"
  [CAN4_Fr_FogLamp] -> bus_creator/34  "CAN4_Fr_FogLamp"
  [CAN4_Fr_Wiper_H] -> bus_creator/35  "CAN4_Fr_Wiper_H"
  [CAN4_Fr_Wiper_L] -> bus_creator/36  "CAN4_Fr_Wiper_L"
  [CAN4_HWResetSta] -> bus_creator/37  "CAN4_HWResetSta"
  [CAN4_H_Beam] -> bus_creator/38  "CAN4_H_Beam"
  [CAN4_H_Beam_ADB] -> bus_creator/39  "CAN4_H_Beam_ADB"
  [CAN4_HazardSW] -> bus_creator/40  "CAN4_HazardSW"
  [CAN4_HoodSW] -> bus_creator/41  "CAN4_HoodSW"
  [CAN4_HornCtrl] -> bus_creator/42  "CAN4_HornCtrl"
  [CAN4_LBSD] -> bus_creator/43  "CAN4_LBSD"
  [CAN4_LDRL] -> bus_creator/44  "CAN4_LDRL"
  [CAN4_LTurnLP] -> bus_creator/45  "CAN4_LTurnLP"
  [CAN4_L_APM_WdwEnable] -> bus_creator/46  "CAN4_L_APM_WdwEnable"
  [CAN4_L_Beam] -> bus_creator/47  "CAN4_L_Beam"
  [CAN4_LampPwr] -> bus_creator/48  "CAN4_LampPwr"
  [CAN4_LockSetting] -> bus_creator/49  "CAN4_LockSetting"
  [CAN4_MSA_Crl_Sta] -> bus_creator/50  "CAN4_MSA_Crl_Sta"
  [CAN4_MirrorCtrl] -> bus_creator/51  "CAN4_MirrorCtrl"
  [CAN4_MirrorDefog] -> bus_creator/52  "CAN4_MirrorDefog"
  [CAN4_PosLamp] -> bus_creator/53  "CAN4_PosLamp"
  [CAN4_PsDoorSW] -> bus_creator/54  "CAN4_PsDoorSW"
  [CAN4_PwrSta] -> bus_creator/55  "CAN4_PwrSta"
  [CAN4_RBSD] -> bus_creator/56  "CAN4_RBSD"
  [CAN4_RC_VCU1_CAN4] -> bus_creator/57  "CAN4_RC_VCU1_CAN4"
  [CAN4_RDRL] -> bus_creator/58  "CAN4_RDRL"
  [CAN4_RLDoorSW] -> bus_creator/59  "CAN4_RLDoorSW"
  [CAN4_RRDoorSW] -> bus_creator/60  "CAN4_RRDoorSW"
  [CAN4_RTurnLP] -> bus_creator/61  "CAN4_RTurnLP"
  [CAN4_ReBrakeLPReq] -> bus_creator/62  "CAN4_ReBrakeLPReq"
  [CAN4_ReverseLamp] -> bus_creator/63  "CAN4_ReverseLamp"
  [CAN4_RoomLampH] -> bus_creator/64  "CAN4_RoomLampH"
  [CAN4_RoomLampL] -> bus_creator/65  "CAN4_RoomLampL"
  [CAN4_Rr_ChargingDoorCtrl] -> bus_creator/66  "CAN4_Rr_ChargingDoorCtrl"
  [CAN4_Rr_Defog] -> bus_creator/67  "CAN4_Rr_Defog"
  [CAN4_Rr_FogLamp] -> bus_creator/68  "CAN4_Rr_FogLamp"
  [CAN4_Rr_Wiper] -> bus_creator/69  "CAN4_Rr_Wiper"
  [CAN4_ShiftGearPosn] -> bus_creator/70  "CAN4_ShiftGearPosn"
  [CAN4_TailgateHDSW] -> bus_creator/71  "CAN4_TailgateHDSW"
  [CAN4_TailgateRemote] -> bus_creator/72  "CAN4_TailgateRemote"
  [CAN4_Tailgate_SW] -> bus_creator/73  "CAN4_Tailgate_SW"
  [CAN4_TimeSNDKCFbk] -> bus_creator/74  "CAN4_TimeSNDKCFbk"
  [CAN4_TrunkRel] -> bus_creator/75  "CAN4_TrunkRel"
  [CAN4_WasherCtrl] -> bus_creator/76  "CAN4_WasherCtrl"
  [CAN4_WiperFixMode] -> bus_creator/77  "CAN4_WiperFixMode"
  bus_creator/1 -> FD4_CE100_0/1
  APSStaSystem/1(CAN4_APS_Sta_System) -> [CAN4_APS_Sta_System]
  AllDoorSW/1(CAN4_AllDoorSW) -> [CAN4_AllDoorSW]
  AntiTheftSeatFold/1(CAN4_AntiTheftSeatFold) -> [CAN4_AntiTheftSeatFold]
  AntitheftSta/1(CAN4_AntitheftSta) -> [CAN4_AntitheftSta]
  BCMDoorLockSta/1(CAN4_BCM_DoorLock_Sta) -> [CAN4_BCM_DoorLock_Sta]
  BrakeLamp/1(CAN4_BrakeLamp) -> [CAN4_BrakeLamp]
  CCCrlSta/1(CAN4_CC_Crl_Sta) -> [CAN4_CC_Crl_Sta]
  CSVCU1CAN4/1(CAN4_CS_VCU1_CAN4) -> [CAN4_CS_VCU1_CAN4]
  CTDCtrl/1(CAN4_CTDCtrl) -> [CAN4_CTDCtrl]
  CTDLockSW/1(CAN4_CTDLockSW) -> [CAN4_CTDLockSW]
  CTDUnlockSW/1(CAN4_CTDUnlockSW) -> [CAN4_CTDUnlockSW]
  CrashDetd/1(CAN4_CrashDetd) -> [CAN4_CrashDetd]
  CtrlDrPwrStbA2/1(CAN4_CtrlDrPwrStbA2) -> [CAN4_CtrlDrPwrStbA2]
  CtrlFrBMSCCUCIR/1(CAN4_CtrlFrBMSCCUCIR) -> [CAN4_CtrlFrBMSCCUCIR]
  CtrlFrEDUINVERTER/1(CAN4_CtrlFrEDUINVERTER) -> [CAN4_CtrlFrEDUINVERTER]
  CtrlFrIRC1/1(CAN4_CtrlFrIRC1) -> [CAN4_CtrlFrIRC1]
  CtrlFrPwrStbA1P/1(CAN4_CtrlFrPwrStbA1P) -> [CAN4_CtrlFrPwrStbA1P]
  DKCAuthSta/1(CAN4_DKCAuthSta) -> [CAN4_DKCAuthSta]
  DKCTimeSN/1(CAN4_DKCTimeSN) -> [CAN4_DKCTimeSN]
  Dimmer/1(CAN4_Dimmer) -> [CAN4_Dimmer]
  DimmerEN/1(CAN4_DimmerEN) -> [CAN4_DimmerEN]
  DoorLockIND/1(CAN4_DoorLockIND) -> [CAN4_DoorLockIND]
  DrDoorSW/1(CAN4_DrDoorSW) -> [CAN4_DrDoorSW]
  DrSeatSta/1(CAN4_Dr_SeatSta) -> [CAN4_Dr_SeatSta]
  EquivAccPedalSWSta/1(CAN4_EquivAccPedalSWSta) -> [CAN4_EquivAccPedalSWSta]
  FDCVMCVehPitchAngleSta/1(CAN4_FDC_VMC_VehPitchAngle_Sta) -> [CAN4_FDC_VMC_VehPitchAngle_Sta]
  FDDKCVehDataErr/1(CAN4_FD_DKC_VehData_Err) -> [CAN4_FD_DKC_VehData_Err]
  FDDKCVehDataSta/1(CAN4_FD_DKC_VehData_Sta) -> [CAN4_FD_DKC_VehData_Sta]
  FDTBOXDTCDataErr/1(CAN4_FD_TBOX_DTCData_Err) -> [CAN4_FD_TBOX_DTCData_Err]
  FDTBOXDTCDataSta/1(CAN4_FD_TBOX_DTCData_Sta) -> [CAN4_FD_TBOX_DTCData_Sta]
  FDTBOXVehDataErr/1(CAN4_FD_TBOX_VehData_Err) -> [CAN4_FD_TBOX_VehData_Err]
  FDTBOXVehDataSta/1(CAN4_FD_TBOX_VehData_Sta) -> [CAN4_FD_TBOX_VehData_Sta]
  FrChargingDoorCtrl/1(CAN4_Fr_ChargingDoorCtrl) -> [CAN4_Fr_ChargingDoorCtrl]
  FrFogLamp/1(CAN4_Fr_FogLamp) -> [CAN4_Fr_FogLamp]
  FrWiperH/1(CAN4_Fr_Wiper_H) -> [CAN4_Fr_Wiper_H]
  FrWiperL/1(CAN4_Fr_Wiper_L) -> [CAN4_Fr_Wiper_L]
  HWResetSta/1(CAN4_HWResetSta) -> [CAN4_HWResetSta]
  HBeam/1(CAN4_H_Beam) -> [CAN4_H_Beam]
  HBeamADB/1(CAN4_H_Beam_ADB) -> [CAN4_H_Beam_ADB]
  HazardSW/1(CAN4_HazardSW) -> [CAN4_HazardSW]
  HoodSW/1(CAN4_HoodSW) -> [CAN4_HoodSW]
  HornCtrl/1(CAN4_HornCtrl) -> [CAN4_HornCtrl]
  LBSD/1(CAN4_LBSD) -> [CAN4_LBSD]
  LDRL/1(CAN4_LDRL) -> [CAN4_LDRL]
  LTurnLP/1(CAN4_LTurnLP) -> [CAN4_LTurnLP]
  LAPMWdwEnable/1(CAN4_L_APM_WdwEnable) -> [CAN4_L_APM_WdwEnable]
  LBeam/1(CAN4_L_Beam) -> [CAN4_L_Beam]
  LampPwr/1(CAN4_LampPwr) -> [CAN4_LampPwr]
  LockSetting/1(CAN4_LockSetting) -> [CAN4_LockSetting]
  MSACrlSta/1(CAN4_MSA_Crl_Sta) -> [CAN4_MSA_Crl_Sta]
  MirrorCtrl/1(CAN4_MirrorCtrl) -> [CAN4_MirrorCtrl]
  MirrorDefog/1(CAN4_MirrorDefog) -> [CAN4_MirrorDefog]
  PosLamp/1(CAN4_PosLamp) -> [CAN4_PosLamp]
  PsDoorSW/1(CAN4_PsDoorSW) -> [CAN4_PsDoorSW]
  PwrSta/1(CAN4_PwrSta) -> [CAN4_PwrSta]
  RBSD/1(CAN4_RBSD) -> [CAN4_RBSD]
  RCVCU1CAN4/1(CAN4_RC_VCU1_CAN4) -> [CAN4_RC_VCU1_CAN4]
  RDRL/1(CAN4_RDRL) -> [CAN4_RDRL]
  RLDoorSW/1(CAN4_RLDoorSW) -> [CAN4_RLDoorSW]
  RRDoorSW/1(CAN4_RRDoorSW) -> [CAN4_RRDoorSW]
  RTurnLP/1(CAN4_RTurnLP) -> [CAN4_RTurnLP]
  ReBrakeLPReq/1(CAN4_ReBrakeLPReq) -> [CAN4_ReBrakeLPReq]
  ReverseLamp/1(CAN4_ReverseLamp) -> [CAN4_ReverseLamp]
  RoomLampH/1(CAN4_RoomLampH) -> [CAN4_RoomLampH]
  RoomLampL/1(CAN4_RoomLampL) -> [CAN4_RoomLampL]
  RrChargingDoorCtrl/1(CAN4_Rr_ChargingDoorCtrl) -> [CAN4_Rr_ChargingDoorCtrl]
  RrDefog/1(CAN4_Rr_Defog) -> [CAN4_Rr_Defog]
  RrFogLamp/1(CAN4_Rr_FogLamp) -> [CAN4_Rr_FogLamp]
  RrWiper/1(CAN4_Rr_Wiper) -> [CAN4_Rr_Wiper]
  ShiftGearPosn/1(CAN4_ShiftGearPosn) -> [CAN4_ShiftGearPosn]
  TailgateHDSW/1(CAN4_TailgateHDSW) -> [CAN4_TailgateHDSW]
  TailgateRemote/1(CAN4_TailgateRemote) -> [CAN4_TailgateRemote]
  TailgateSW/1(CAN4_Tailgate_SW) -> [CAN4_Tailgate_SW]
  TimeSNDKCFbk/1(CAN4_TimeSNDKCFbk) -> [CAN4_TimeSNDKCFbk]
  TrunkRel/1(CAN4_TrunkRel) -> [CAN4_TrunkRel]
  WasherCtrl/1(CAN4_WasherCtrl) -> [CAN4_WasherCtrl]
  WiperFixMode/1(CAN4_WiperFixMode) -> [CAN4_WiperFixMode]
  Byte_0/1(Byte_0) -> Terminator/1
  Byte_1/1(Byte_1) -> [Byte_1]
  Byte_2/1(Byte_2) -> [Byte_2]
  Byte_3/1(Byte_3) -> [Byte_3]
  Byte_4/1(Byte_4) -> [Byte_4]
  Byte_5/1(Byte_5) -> [Byte_5]
  Byte_6/1(Byte_6) -> [Byte_6]
  Byte_7/1(Byte_7) -> [Byte_7]
  Byte_8/1(Byte_8) -> [Byte_8]
  Byte_9/1(Byte_9) -> [Byte_9]
  Byte_10/1(Byte_10) -> [Byte_10]
  Byte_11/1(Byte_11) -> [Byte_11]
  Byte_12/1(Byte_12) -> [Byte_12]
  Byte_13/1(Byte_13) -> [Byte_13]
  Byte_14/1(Byte_14) -> [Byte_14]
  Byte_15/1(Byte_15) -> [Byte_15]
  Byte_16/1(Byte_16) -> [Byte_16]
  Byte_17/1(Byte_17) -> [Byte_17]
  Byte_18/1 -> [Byte_18]
  Byte_19/1(Byte_19) -> [Byte_19]
  Byte_20/1(Byte_20) -> [Byte_20]
  Byte_21/1(Byte_21) -> [Byte_21]
  Byte_22/1(Byte_22) -> [Byte_22]
  Byte_23/1(Byte_23) -> [Byte_23]
  Byte_24/1 -> [Byte_24]
  Byte_25/1(Byte_25) -> [Byte_25]
  Byte_26/1(Byte_26) -> [Byte_26]
  Byte_27/1(Byte_27) -> [Byte_27]
  Byte_28/1 -> [Byte_28]
  Byte_29/1 -> [Byte_29]
  Byte_30/1 -> [Byte_30]
  Byte_31/1 -> [Byte_31]
  Mux2/1 -> CRC8_IfAction_Tx/4(RawData)
  Constant/1 -> CRC8_IfAction_Tx/1(CAN_E2E_flg)
  Constant1/1 -> CRC8_IfAction_Tx/2(DataID1)
  Constant2/1 -> CRC8_IfAction_Tx/3(DataID2)
  CRC8_IfAction_Tx/1(CRC8) -> [CS_VCU1_CAN4]
  Ground/1 -> Byte_0/1(CS_VCU1_CAN4)
  [Byte_1] -> Mux2/1
  RollingCounter_IfAction/1 -> Byte_1/1(RC_VCU1_CAN4)
  Constant3/1 -> RollingCounter_IfAction/1
  [Byte_2] -> Mux2/2
  bus_selector/1 -> Byte_2/1(CC_Crl_Sta)  "<VOUTP_CCCtrlSta_enum>"
  [BOUTP_outputs] -> bus_selector/1
  bus_selector1/1 -> Byte_2/2(Dr_SeatSta)  "<VOUTP_DrSeatSta_enum>"
  [BOUTP_outputs] -> bus_selector1/1
  bus_selector2/1 -> Byte_2/3(MSA_Crl_Sta)  "<VOUTP_MSACtrlSta_enum>"
  [BOUTP_outputs] -> bus_selector2/1
  [Byte_3] -> Mux2/3
  bus_selector4/1 -> Byte_3/2(PwrSta)  "<VOUTP_PowerSta_enum>"
  [BOUTP_outputs] -> bus_selector4/1
  bus_selector5/1 -> Byte_3/3(ReBrakeLPReq)  "<VOUTP_ReBrakeLPReq_flg>"
  [BOUTP_outputs] -> bus_selector5/1
  bus_selector6/1 -> Byte_3/4(ShiftGearPosn)  "<VOUTP_ShiftGearPosn_enum>"
  [BOUTP_outputs] -> bus_selector6/1
  [Byte_4] -> Mux2/4
  bus_selector7/1 -> Byte_4/1(DKCTimeSN)  "<VOUTP_DKCTimeSN_cnt>"
  [BOUTP_outputs] -> bus_selector7/1
  [Byte_5] -> Mux2/5
  bus_selector8/1 -> Byte_5/1(DKCTimeSN)  "<VOUTP_DKCTimeSN_cnt>"
  [BOUTP_outputs] -> bus_selector8/1
  [Byte_6] -> Mux2/6
  bus_selector9/1 -> Byte_6/1(DKCTimeSN)  "<VOUTP_DKCTimeSN_cnt>"
  [BOUTP_outputs] -> bus_selector9/1
  [Byte_7] -> Mux2/7
  bus_selector10/1 -> Byte_7/1(DKCTimeSN)  "<VOUTP_DKCTimeSN_cnt>"
  [BOUTP_outputs] -> bus_selector10/1
  [Byte_8] -> Mux2/8
  Ground1/1 -> Byte_8/1(TimeSNDKCFbk)
  [Byte_9] -> Mux2/9
  Ground2/1 -> Byte_9/1(TimeSNDKCFbk)
  [Byte_10] -> Mux2/10
  Ground3/1 -> Byte_10/1(TimeSNDKCFbk)
  [Byte_11] -> Mux2/11
  Ground4/1 -> Byte_11/1(TimeSNDKCFbk)
  [Byte_12] -> Mux2/12
  bus_selector11/1 -> Byte_12/1(BCM_DoorLock_Sta)  "<VOUTP_BCMDoorLockSta_flg>"
  [BOUTP_outputs] -> bus_selector11/1
  bus_selector12/1 -> Byte_12/2(DimmerEN)  "<VOUTP_DimmerEN_flg>"
  [BOUTP_outputs] -> bus_selector12/1
  bus_selector13/1 -> Byte_12/3(EquivAccPedalSWSta)  "<VOUTP_EquivAccPedalSWSta_flg>"
  [BOUTP_outputs] -> bus_selector13/1
  bus_selector14/1 -> Byte_12/4(HornCtrl)  "<VOUTP_HornCtrl_flg>"
  [BOUTP_outputs] -> bus_selector14/1
  bus_selector15/1 -> Byte_12/5(RoomLampH)  "<VOUTP_RoomLampH_flg>"
  [BOUTP_outputs] -> bus_selector15/1
  bus_selector16/1 -> Byte_12/6(RoomLampL)  "<VOUTP_RoomLampL_flg>"
  [BOUTP_outputs] -> bus_selector16/1
  bus_selector17/1 -> Byte_12/7(TailgateRemote)  "<VOUTP_TailgateRemote_enum>"
  [BOUTP_outputs] -> bus_selector17/1
  [Byte_13] -> Mux2/13
  bus_selector18/1 -> Byte_13/1(Dimmer)  "<VOUTP_Dimmer_pct>"
  [BOUTP_outputs] -> bus_selector18/1
  [Byte_14] -> Mux2/14
  bus_selector19/1 -> Byte_14/1(AntiTheftSeatFold)  "<VOUTP_AntitheftSeatFlod_flg>"
  [BOUTP_outputs] -> bus_selector19/1
  bus_selector20/1 -> Byte_14/2(AntitheftSta)  "<VOUTP_AntitheftSta_enum>"
  [BOUTP_outputs] -> bus_selector20/1
  bus_selector21/1 -> Byte_14/3(CrashDetd)  "<VOUTP_CrashDetd_flg>"
  [BOUTP_outputs] -> bus_selector21/1
  Ground5/1 -> Byte_14/4(L_APM_WdwEnable)
  bus_selector22/1 -> Byte_14/5(LockSetting)  "<VOUTP_LockSetting_flg>"
  [BOUTP_outputs] -> bus_selector22/1
  bus_selector23/1 -> Byte_14/6(RTurnLP)  "<VOUTP_RTurnLP_flg>"
  [BOUTP_outputs] -> bus_selector23/1
  [Byte_15] -> Mux2/15
  bus_selector24/1 -> Byte_15/1(BrakeLamp)  "<VOUTP_BrakeLamp_flg>"
  [BOUTP_outputs] -> bus_selector24/1
  Ground6/1 -> Byte_15/2(Fr_FogLamp)
  bus_selector25/1 -> Byte_15/3(HazardSW)  "<VOUTP_HazardSW_flg>"
  [BOUTP_outputs] -> bus_selector25/1
  bus_selector26/1 -> Byte_15/4(LBSD)  "<VOUTP_LBSD_flg>"
  [BOUTP_outputs] -> bus_selector26/1
  bus_selector27/1 -> Byte_15/5(LTurnLP)  "<VOUTP_LTurnLP_flg>"
  [BOUTP_outputs] -> bus_selector27/1
  bus_selector28/1 -> Byte_15/6(RBSD)  "<VOUTP_RBSD_flg>"
  [BOUTP_outputs] -> bus_selector28/1
  bus_selector29/1 -> Byte_15/7(ReverseLamp)  "<VOUTP_ReverseLamp_flg>"
  [BOUTP_outputs] -> bus_selector29/1
  bus_selector30/1 -> Byte_15/8(Rr_FogLamp)  "<VOUTP_RrFogLamp_flg>"
  [BOUTP_outputs] -> bus_selector30/1
  [Byte_16] -> Mux2/16
  bus_selector31/1 -> Byte_16/1(H_Beam)  "<VOUTP_HBeam_flg>"
  [BOUTP_outputs] -> bus_selector31/1
  bus_selector32/1 -> Byte_16/2(LDRL)  "<VOUTP_LDRL_flg>"
  [BOUTP_outputs] -> bus_selector32/1
  bus_selector33/1 -> Byte_16/3(L_Beam)  "<VOUTP_LBeam_flg>"
  [BOUTP_outputs] -> bus_selector33/1
  bus_selector34/1 -> Byte_16/4(PosLamp)  "<VOUTP_PosLamp_flg>"
  [BOUTP_outputs] -> bus_selector34/1
  bus_selector35/1 -> Byte_16/5(RDRL)  "<VOUTP_RDRL_flg>"
  [BOUTP_outputs] -> bus_selector35/1
  bus_selector36/1 -> Byte_16/6(WasherCtrl)  "<VOUTP_WasherCtrl_enum>"
  [BOUTP_outputs] -> bus_selector36/1
  bus_selector37/1 -> Byte_16/7(WiperFixMode)  "<VOUTP_WiperFixMode_flg>"
  [BOUTP_outputs] -> bus_selector37/1
  [Byte_17] -> Mux2/17
  bus_selector38/1 -> Byte_17/1(Fr_Wiper_H)  "<VOUTP_FrWiperH_flg>"
  [BOUTP_outputs] -> bus_selector38/1
  bus_selector39/1 -> Byte_17/2(Fr_Wiper_L)  "<VOUTP_FrWiperL_flg>"
  [BOUTP_outputs] -> bus_selector39/1
  bus_selector40/1 -> Byte_17/3(MirrorCtrl)  "<VOUTP_MirrorCtrl_enum>"
  [BOUTP_outputs] -> bus_selector40/1
  bus_selector41/1 -> Byte_17/4(Rr_Defog)  "<VOUTP_RrDefog_flg>"
  [BOUTP_outputs] -> bus_selector41/1
  bus_selector42/1 -> Byte_17/5(Rr_Wiper)  "<VOUTP_RrWiper_flg>"
  [BOUTP_outputs] -> bus_selector42/1
  bus_selector43/1 -> Byte_17/6(TailgateHDSW)  "<VOUTP_TailgateHDSW_flg>"
  [BOUTP_outputs] -> bus_selector43/1
  bus_selector44/1 -> Byte_17/7(TrunkRel)  "<VOUTP_TrunkRel_flg>"
  [BOUTP_outputs] -> bus_selector44/1
  [Byte_18] -> Mux2/18
  [Byte_19] -> Mux2/19
  bus_selector45/1 -> Byte_19/1(AllDoorSW)  "<VOUTP_AllDoorSW_flg>"
  [BOUTP_outputs] -> bus_selector45/1
  bus_selector46/1 -> Byte_19/2(DoorLockIND)  "<VOUTP_DoorLockIND_flg>"
  [BOUTP_outputs] -> bus_selector46/1
  bus_selector47/1 -> Byte_19/3(Fr_ChargingDoorCtrl)  "<VOUTP_FrChargingDoorCtrl_enum>"
  [BOUTP_outputs] -> bus_selector47/1
  bus_selector48/1 -> Byte_19/4(HoodSW)  "<VOUTP_HoodSW_flg>"
  [BOUTP_outputs] -> bus_selector48/1
  bus_selector49/1 -> Byte_19/5(PsDoorSW)  "<VOUTP_PsDoorSW_flg>"
  [BOUTP_outputs] -> bus_selector49/1
  bus_selector50/1 -> Byte_19/6(RLDoorSW)  "<VOUTP_RLDoorSW_flg>"
  [BOUTP_outputs] -> bus_selector50/1
  bus_selector51/1 -> Byte_19/7(RRDoorSW)  "<VOUTP_RRDoorSW_flg>"
  [BOUTP_outputs] -> bus_selector51/1
  [Byte_20] -> Mux2/20
  bus_selector52/1 -> Byte_20/1(CTDCtrl)  "<VOUTP_CTDCtrl_enum>"
  [BOUTP_outputs] -> bus_selector52/1
  Ground7/1 -> Byte_20/2(FD_TBOX_VehData_Sta)
  bus_selector53/1 -> Byte_20/3(Rr_ChargingDoorCtrl)  "<VOUTP_RrChargingDoorCtrl_enum>"
  [BOUTP_outputs] -> bus_selector53/1
  [Byte_21] -> Mux2/21
  Ground8/1 -> Byte_21/1(FD_DKC_VehData_Sta)
  Ground9/1 -> Byte_21/2(FD_TBOX_VehData_Err)
  [Byte_22] -> Mux2/22
  Ground10/1 -> Byte_22/1(FD_DKC_VehData_Err)
  Ground11/1 -> Byte_22/2(FD_TBOX_DTCData_Sta)
  [Byte_23] -> Mux2/23
  bus_selector54/1 -> Byte_23/1(DKCAuthSta)  "<VOUTP_DKCAuthSta_enum>"
  [BOUTP_outputs] -> bus_selector54/1
  Ground12/1 -> Byte_23/2(FD_TBOX_DTCData_Err)
  bus_selector55/1 -> Byte_23/3(LampPwr)  "<VOUTP_LampPwr_flg>"
  [BOUTP_outputs] -> bus_selector55/1
  [Byte_24] -> Mux2/24
  [Byte_25] -> Mux2/25
  bus_selector56/1 -> Byte_25/1(CtrlFrBMSCCUCIR)  "<VOUTP_CtrlFrBMSCCUCIR_flg>"
  [BOUTP_outputs] -> bus_selector56/1
  bus_selector57/1 -> Byte_25/2(CtrlFrEDUINVERTER)  "<VOUTP_CtrlFrEDUINVERTER_flg>"
  [BOUTP_outputs] -> bus_selector57/1
  bus_selector58/1 -> Byte_25/3(CtrlFrIRC1)  "<VOUTP_CtrlFrRC1_flg>"
  [BOUTP_outputs] -> bus_selector58/1
  bus_selector59/1 -> Byte_25/4(CtrlFrPwrStbA1P)  "<VOUTP_CtrlFrPwrStbA1P_flg>"
  [BOUTP_outputs] -> bus_selector59/1
  bus_selector60/1 -> Byte_25/5(DrDoorSW)  "<VOUTP_DrDoorSW_flg>"
  [BOUTP_outputs] -> bus_selector60/1
  bus_selector61/1 -> Byte_25/6(HWResetSta)  "<VOUTP_HWResetSta_enum>"
  [BOUTP_outputs] -> bus_selector61/1
  bus_selector62/1 -> Byte_25/7(MirrorDefog)  "<VOUTP_MirrorDefog_flg>"
  [BOUTP_outputs] -> bus_selector62/1
  [Byte_26] -> Mux2/26
  bus_selector63/1 -> Byte_26/1(APS_Sta_System)  "<VOUTP_APSStaSys_enum>"
  [BOUTP_outputs] -> bus_selector63/1
  bus_selector64/1 -> Byte_26/2(CTDLockSW)  "<VOUTP_CTDLockSW_flg>"
  [BOUTP_outputs] -> bus_selector64/1
  Ground13/1 -> Byte_26/3(CTDUnlockSW)
  bus_selector65/1 -> Byte_26/4(FDC_VMC_VehPitchAngle_Sta)  "<VOUTP_VehPitchAngleSta_enum>"
  [BOUTP_outputs] -> bus_selector65/1
  [Byte_27] -> Mux2/27
  bus_selector66/1 -> Byte_27/1(CtrlDrPwrStbA2)  "<VOUTP_CtrlDrPwrStbA2_flg>"
  [BOUTP_outputs] -> bus_selector66/1
  bus_selector67/1 -> Byte_27/2(Tailgate_SW)  "<VOUTP_TailgateSW_flg>"
  [BOUTP_outputs] -> bus_selector67/1
  bus_selector68/1 -> APSStaSystem/1(APSStaSystem)  "<VOUTP_APSStaSys_enum>"
  [BOUTP_outputs] -> bus_selector68/1
  bus_selector69/1 -> AllDoorSW/1(AllDoorSW)  "<VOUTP_AllDoorSW_flg>"
  [BOUTP_outputs] -> bus_selector69/1
  bus_selector70/1 -> AntiTheftSeatFold/1(AntiTheftSeatFold)  "<VOUTP_AntitheftSeatFlod_flg>"
  [BOUTP_outputs] -> bus_selector70/1
  bus_selector71/1 -> AntitheftSta/1(AntitheftSta)  "<VOUTP_AntitheftSta_enum>"
  [BOUTP_outputs] -> bus_selector71/1
  bus_selector72/1 -> BCMDoorLockSta/1(BCMDoorLockSta)  "<VOUTP_BCMDoorLockSta_flg>"
  [BOUTP_outputs] -> bus_selector72/1
  bus_selector73/1 -> BrakeLamp/1(BrakeLamp)  "<VOUTP_BrakeLamp_flg>"
  [BOUTP_outputs] -> bus_selector73/1
  bus_selector74/1 -> CCCrlSta/1(CCCrlSta)  "<VOUTP_CCCtrlSta_enum>"
  [BOUTP_outputs] -> bus_selector74/1
  [CS_VCU1_CAN4] -> CSVCU1CAN4/1(CSVCU1CAN4)
  bus_selector75/1 -> CTDCtrl/1(CTDCtrl)  "<VOUTP_CTDCtrl_enum>"
  [BOUTP_outputs] -> bus_selector75/1
  bus_selector76/1 -> CTDLockSW/1(CTDLockSW)  "<VOUTP_CTDLockSW_flg>"
  [BOUTP_outputs] -> bus_selector76/1
  Ground14/1 -> CTDUnlockSW/1(CTDUnlockSW)
  bus_selector77/1 -> CrashDetd/1(CrashDetd)  "<VOUTP_CrashDetd_flg>"
  [BOUTP_outputs] -> bus_selector77/1
  bus_selector78/1 -> CtrlDrPwrStbA2/1(CtrlDrPwrStbA2)  "<VOUTP_CtrlDrPwrStbA2_flg>"
  [BOUTP_outputs] -> bus_selector78/1
  bus_selector79/1 -> CtrlFrBMSCCUCIR/1(CtrlFrBMSCCUCIR)  "<VOUTP_CtrlFrBMSCCUCIR_flg>"
  [BOUTP_outputs] -> bus_selector79/1
  bus_selector80/1 -> CtrlFrEDUINVERTER/1(CtrlFrEDUINVERTER)  "<VOUTP_CtrlFrEDUINVERTER_flg>"
  [BOUTP_outputs] -> bus_selector80/1
  bus_selector81/1 -> CtrlFrIRC1/1(CtrlFrIRC1)  "<VOUTP_CtrlFrRC1_flg>"
  [BOUTP_outputs] -> bus_selector81/1
  bus_selector82/1 -> CtrlFrPwrStbA1P/1(CtrlFrPwrStbA1P)  "<VOUTP_CtrlFrPwrStbA1P_flg>"
  [BOUTP_outputs] -> bus_selector82/1
  bus_selector83/1 -> DKCAuthSta/1(DKCAuthSta)  "<VOUTP_DKCAuthSta_enum>"
  [BOUTP_outputs] -> bus_selector83/1
  bus_selector84/1 -> DKCTimeSN/1(DKCTimeSN)  "<VOUTP_DKCTimeSN_cnt>"
  [BOUTP_outputs] -> bus_selector84/1
  bus_selector85/1 -> Dimmer/1(Dimmer)  "<VOUTP_Dimmer_pct>"
  [BOUTP_outputs] -> bus_selector85/1
  bus_selector86/1 -> DimmerEN/1(DimmerEN)  "<VOUTP_DimmerEN_flg>"
  [BOUTP_outputs] -> bus_selector86/1
  bus_selector87/1 -> DoorLockIND/1(DoorLockIND)  "<VOUTP_DoorLockIND_flg>"
  [BOUTP_outputs] -> bus_selector87/1
  bus_selector88/1 -> DrDoorSW/1(DrDoorSW)  "<VOUTP_DrDoorSW_flg>"
  [BOUTP_outputs] -> bus_selector88/1
  bus_selector89/1 -> DrSeatSta/1(DrSeatSta)  "<VOUTP_DrSeatSta_enum>"
  [BOUTP_outputs] -> bus_selector89/1
  bus_selector90/1 -> EquivAccPedalSWSta/1(EquivAccPedalSWSta)  "<VOUTP_EquivAccPedalSWSta_flg>"
  [BOUTP_outputs] -> bus_selector90/1
  bus_selector91/1 -> FDCVMCVehPitchAngleSta/1(FDCVMCVehPitchAngleSta)  "<VOUTP_VehPitchAngleSta_enum>"
  [BOUTP_outputs] -> bus_selector91/1
  Ground15/1 -> FDDKCVehDataErr/1(FDDKCVehDataErr)
  Ground16/1 -> FDDKCVehDataSta/1(FDDKCVehDataSta)
  Ground17/1 -> FDTBOXDTCDataErr/1(FDTBOXDTCDataErr)
  Ground18/1 -> FDTBOXDTCDataSta/1(FDTBOXDTCDataSta)
  Ground19/1 -> FDTBOXVehDataErr/1(FDTBOXVehDataErr)
  Ground20/1 -> FDTBOXVehDataSta/1(FDTBOXVehDataSta)
  bus_selector92/1 -> FrChargingDoorCtrl/1(FrChargingDoorCtrl)  "<VOUTP_FrChargingDoorCtrl_enum>"
  [BOUTP_outputs] -> bus_selector92/1
  Ground21/1 -> FrFogLamp/1(FrFogLamp)
  bus_selector93/1 -> FrWiperH/1(FrWiperH)  "<VOUTP_FrWiperH_flg>"
  [BOUTP_outputs] -> bus_selector93/1
  bus_selector94/1 -> FrWiperL/1(FrWiperL)  "<VOUTP_FrWiperL_flg>"
  [BOUTP_outputs] -> bus_selector94/1
  bus_selector95/1 -> HWResetSta/1(HWResetSta)  "<VOUTP_HWResetSta_enum>"
  [BOUTP_outputs] -> bus_selector95/1
  bus_selector96/1 -> HBeam/1(HBeam)  "<VOUTP_HBeam_flg>"
  [BOUTP_outputs] -> bus_selector96/1
  bus_selector98/1 -> HazardSW/1(HazardSW)  "<VOUTP_HazardSW_flg>"
  [BOUTP_outputs] -> bus_selector98/1
  bus_selector99/1 -> HoodSW/1(HoodSW)  "<VOUTP_HoodSW_flg>"
  [BOUTP_outputs] -> bus_selector99/1
  bus_selector100/1 -> HornCtrl/1(HornCtrl)  "<VOUTP_HornCtrl_flg>"
  [BOUTP_outputs] -> bus_selector100/1
  bus_selector101/1 -> LBSD/1(LBSD)  "<VOUTP_LBSD_flg>"
  [BOUTP_outputs] -> bus_selector101/1
  bus_selector102/1 -> LDRL/1(LDRL)  "<VOUTP_LDRL_flg>"
  [BOUTP_outputs] -> bus_selector102/1
  bus_selector103/1 -> LTurnLP/1(LTurnLP)  "<VOUTP_LTurnLP_flg>"
  [BOUTP_outputs] -> bus_selector103/1
  Ground22/1 -> LAPMWdwEnable/1(LAPMWdwEnable)
  bus_selector104/1 -> LBeam/1(LBeam)  "<VOUTP_LBeam_flg>"
  [BOUTP_outputs] -> bus_selector104/1
  bus_selector105/1 -> LampPwr/1(LampPwr)  "<VOUTP_LampPwr_flg>"
  [BOUTP_outputs] -> bus_selector105/1
  bus_selector106/1 -> LockSetting/1(LockSetting)  "<VOUTP_LockSetting_flg>"
  [BOUTP_outputs] -> bus_selector106/1
  bus_selector107/1 -> MSACrlSta/1(MSACrlSta)  "<VOUTP_MSACtrlSta_enum>"
  [BOUTP_outputs] -> bus_selector107/1
  bus_selector108/1 -> MirrorCtrl/1(MirrorCtrl)  "<VOUTP_MirrorCtrl_enum>"
  [BOUTP_outputs] -> bus_selector108/1
  bus_selector109/1 -> MirrorDefog/1(MirrorDefog)  "<VOUTP_MirrorDefog_flg>"
  [BOUTP_outputs] -> bus_selector109/1
  bus_selector110/1 -> PosLamp/1(PosLamp)  "<VOUTP_PosLamp_flg>"
  [BOUTP_outputs] -> bus_selector110/1
  bus_selector111/1 -> PsDoorSW/1(PsDoorSW)  "<VOUTP_PsDoorSW_flg>"
  [BOUTP_outputs] -> bus_selector111/1
  bus_selector112/1 -> PwrSta/1(PwrSta)  "<VOUTP_PowerSta_enum>"
  [BOUTP_outputs] -> bus_selector112/1
  bus_selector113/1 -> RBSD/1(RBSD)  "<VOUTP_RBSD_flg>"
  [BOUTP_outputs] -> bus_selector113/1
  RollingCounter_IfAction1/1 -> RCVCU1CAN4/1(RCVCU1CAN4)
  Constant4/1 -> RollingCounter_IfAction1/1
  bus_selector114/1 -> RDRL/1(RDRL)  "<VOUTP_RDRL_flg>"
  [BOUTP_outputs] -> bus_selector114/1
  bus_selector115/1 -> RLDoorSW/1(RLDoorSW)  "<VOUTP_RLDoorSW_flg>"
  [BOUTP_outputs] -> bus_selector115/1
  bus_selector116/1 -> RRDoorSW/1(RRDoorSW)  "<VOUTP_RRDoorSW_flg>"
  [BOUTP_outputs] -> bus_selector116/1
  bus_selector117/1 -> RTurnLP/1(RTurnLP)  "<VOUTP_RTurnLP_flg>"
  [BOUTP_outputs] -> bus_selector117/1
  bus_selector118/1 -> ReBrakeLPReq/1(ReBrakeLPReq)  "<VOUTP_ReBrakeLPReq_flg>"
  [BOUTP_outputs] -> bus_selector118/1
  bus_selector119/1 -> ReverseLamp/1(ReverseLamp)  "<VOUTP_ReverseLamp_flg>"
  [BOUTP_outputs] -> bus_selector119/1
  bus_selector120/1 -> RoomLampH/1(RoomLampH)  "<VOUTP_RoomLampH_flg>"
  [BOUTP_outputs] -> bus_selector120/1
  bus_selector121/1 -> RoomLampL/1(RoomLampL)  "<VOUTP_RoomLampL_flg>"
  [BOUTP_outputs] -> bus_selector121/1
  bus_selector122/1 -> RrChargingDoorCtrl/1(RrChargingDoorCtrl)  "<VOUTP_RrChargingDoorCtrl_enum>"
  [BOUTP_outputs] -> bus_selector122/1
  bus_selector123/1 -> RrDefog/1(RrDefog)  "<VOUTP_RrDefog_flg>"
  [BOUTP_outputs] -> bus_selector123/1
  bus_selector124/1 -> RrFogLamp/1(RrFogLamp)  "<VOUTP_RrFogLamp_flg>"
  [BOUTP_outputs] -> bus_selector124/1
  bus_selector125/1 -> RrWiper/1(RrWiper)  "<VOUTP_RrWiper_flg>"
  [BOUTP_outputs] -> bus_selector125/1
  bus_selector126/1 -> ShiftGearPosn/1(ShiftGearPosn)  "<VOUTP_ShiftGearPosn_enum>"
  [BOUTP_outputs] -> bus_selector126/1
  bus_selector127/1 -> TailgateHDSW/1(TailgateHDSW)  "<VOUTP_TailgateHDSW_flg>"
  [BOUTP_outputs] -> bus_selector127/1
  bus_selector128/1 -> TailgateRemote/1(TailgateRemote)  "<VOUTP_TailgateRemote_enum>"
  [BOUTP_outputs] -> bus_selector128/1
  bus_selector129/1 -> TailgateSW/1(TailgateSW)  "<VOUTP_TailgateSW_flg>"
  [BOUTP_outputs] -> bus_selector129/1
  Ground23/1 -> TimeSNDKCFbk/1(TimeSNDKCFbk)
  bus_selector130/1 -> TrunkRel/1(TrunkRel)  "<VOUTP_TrunkRel_flg>"
  [BOUTP_outputs] -> bus_selector130/1
  bus_selector131/1 -> WasherCtrl/1(WasherCtrl)  "<VOUTP_WasherCtrl_enum>"
  [BOUTP_outputs] -> bus_selector131/1
  bus_selector132/1 -> WiperFixMode/1(WiperFixMode)  "<VOUTP_WiperFixMode_flg>"
  [BOUTP_outputs] -> bus_selector132/1
  Ground24/1 -> Byte_3/1(H_Beam_ADB)
  Ground25/1 -> HBeamADB/1(HBeamADB)
